simulink model "ObserverDesign"  (R2023a)
settings: Solver=VariableStepAuto  StartTime=0.0  StopTime=10.0  RelTol=1e-3
settings Model: Creator=19591  LastModifiedBy=19591

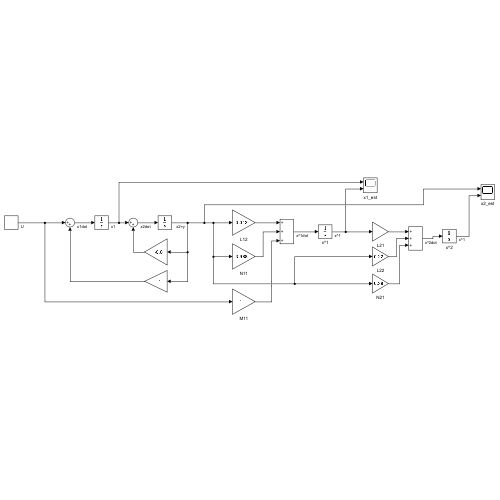
[thumbnail: Simulink's stored preview of the top-level diagram]
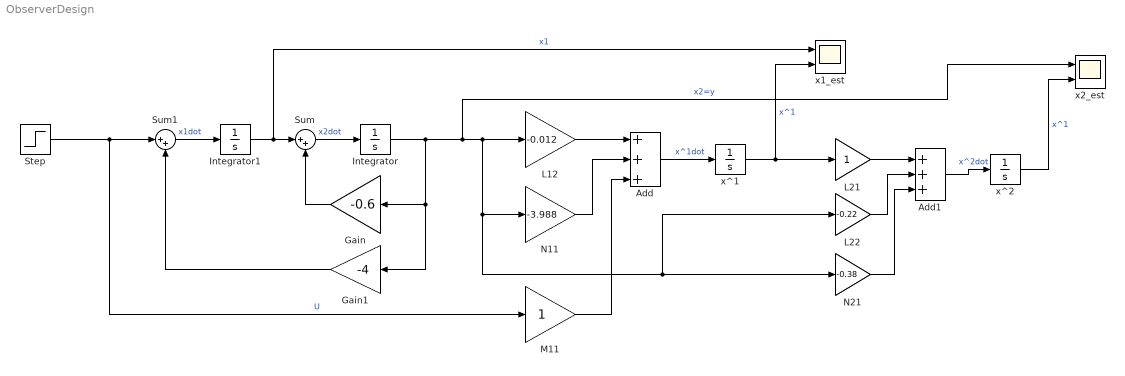
== system ObserverDesign ==
  Add : Sum  Inputs=+++
  Add1 : Sum  Inputs=+++
  Gain : Gain  Gain=-0.6
  Gain1 : Gain  Gain=-4
  Integrator : Integrator
  Integrator1 : Integrator
  L12 : Gain  Gain=-0.012
  L21 : Gain
  L22 : Gain  Gain=-0.22
  M11 : Gain
  N11 : Gain  Gain=-3.988
  N21 : Gain  Gain=-0.38
  Step : Step  SampleTime=0
  Sum : Sum  Inputs=|++
  Sum1 : Sum  Inputs=|++
  x1_est : Scope  NumInputPorts=2
  x2_est : Scope  NumInputPorts=2
  x^1 : Integrator
  x^2 : Integrator
  wires:
  Sum1/1 -> Integrator1/1  "x1dot"
  Integrator/1 -> x2_est/1, L22/1, N21/1, N11/1, L12/1, Gain1/1, Gain/1  "x2=y"
  Gain1/1 -> Sum1/2
  Integrator1/1 -> x1_est/1, Sum/1  "x1"
  Gain/1 -> Sum/2
  Sum/1 -> Integrator/1  "x2dot"
  Step/1 -> M11/1, Sum1/1  "U"
  L12/1 -> Add/1
  N11/1 -> Add/2
  M11/1 -> Add/3
  Add/1 -> x^1/1  "x^1dot"
  x^1/1 -> x1_est/2, L21/1  "x^1"
  L21/1 -> Add1/1
  L22/1 -> Add1/2
  N21/1 -> Add1/3
  Add1/1 -> x^2/1  "x^2dot"
  x^2/1 -> x2_est/2  "x^1"
